simulink model "lab4_2"  (R2015a)
settings: Solver=ode5  StartTime=0.0  StopTime=inf  RelTol=1e-3
undefined symbols (not defined in the file or in its folder): National_Instruments, PCI
libraries: rtwinlib x2
settings Model: SimulationMode=external  ExtModeTrigDuration=10000  Creator=u_labelectro  LastModifiedBy=ARTURO
settings DebuggingCC: UnderspecifiedInitializationDetection=Classic  MergeDetectMultiDrivingBlocksExec=none  SolverPrmCheckMsg=warning  StateNameClashWarn=warning
settings HardwareCC: ProdBitPerLong=64  ProdBitPerPointer=64  ProdIntDivRoundTo=Zero  ProdEndianess=LittleEndian  ProdWordSize=64  ProdHWDeviceType=Intel->x86-64  TargetBitPerLong=64  TargetBitPerPointer=64  TargetIntDivRoundTo=Zero  TargetEndianess=LittleEndian  TargetWordSize=64  TargetHWDeviceType=Intel->x86-64
settings RTWCC: SystemTargetFile=rtwin.tlc  TemplateMakefile=rtwin.tmf  Description=Real-Time Windows Target  RTWCompilerOptimization=on
settings CodeAppCC: MaxIdLength=95
settings RTWinTargetCC: TargetPreCompLibLocation=C:\Program Files\MATLAB\MATLAB Production Server\R2015a\toolbox\sldrt\lib\win64

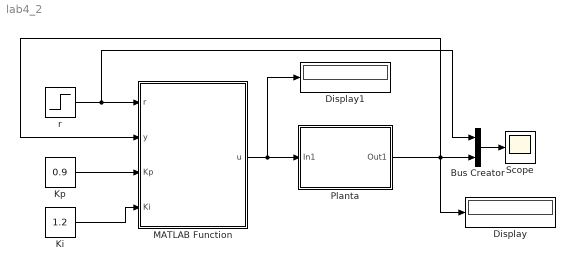
== system lab4_2 ==
  Bus Creator : BusCreator  Inputs=2
  Display : Display
  Display1 : Display
  Ki : Constant  Value=1.2
  Kp : Constant  Value=0.9
  MATLAB Function : MATLAB Function  TreatAsAtomicUnit=on
  Planta : Subsystem
  Scope : Scope
      settings: YMin=0  YMax=120  SaveName=signals
  r : Step  Time=0  After=60  SampleTime=0.01
  wires:
  Kp/1 -> MATLAB Function/3(Kp)
  Ki/1 -> MATLAB Function/4(Ki)
  r/1 -> Bus Creator/1, MATLAB Function/1(r)
  Planta/1(Out1) -> Bus Creator/2, Display/1, MATLAB Function/2(y)
  MATLAB Function/1(u) -> Display1/1, Planta/1(In1)
  Bus Creator/1 -> Scope/1

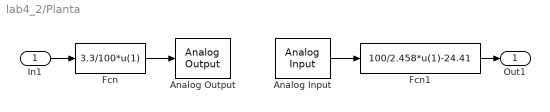
== system lab4_2/Planta ==
  In1 : Inport
  Analog Input : rtwinlib/Analog Input  SampleTime=0.01  MaxMissedTicks=10  ShowMissedTicks=off  YieldWhenWaiting=off  DrvName=National_Instruments/PCI-6229  DrvAddress=4294967295  DrvOptions=[0 0 0 0 0]  Channels=1  RangeMode=1  VoltRange=1  DataType=1
      settings: AttributesFormatString=National Instruments\nPCI-6229 [auto]
  Analog Output : rtwinlib/Analog Output  SampleTime=0.01  MaxMissedTicks=10  ShowMissedTicks=off  YieldWhenWaiting=off  DrvName=National_Instruments/PCI-6229  DrvAddress=4294967295  DrvOptions=[0 0 0 0 0]  Channels=1  RangeMode=1  VoltRange=1  InitialValue=[]  FinalValue=[]
      settings: AttributesFormatString=National Instruments\nPCI-6229 [auto]
  Fcn : Fcn  Expr=3.3/100*u(1)  SampleTime=0.01
  Fcn1 : Fcn  Expr=100/2.458*u(1)-24.41  SampleTime=0.01
  Out1 : Outport
  wires:
  Fcn/1 -> Analog Output/1
  In1/1 -> Fcn/1
  Fcn1/1 -> Out1/1
  Analog Input/1 -> Fcn1/1

== matlab function lab4_2/MATLAB Function ==
  data: r input; y input; Kp input; Ki input; u output
function u = controlador_PI(r,y,Kp,Ki)

T = 0.01;

persistent e_ant;
persistent u_ant;
persistent Int_ant;

if isempty(u_ant)
    u_ant = 0;
    e_ant = 0;
    Int_ant = 0;
end

e_act = r - y;

% Diferencias en retroceso
% Prop = (e_act - e_ant)*Kp;
% Int = e_act*Ki*T;
% u_act = u_ant + Prop + Int;
% Kp = 0.9, Ki = 1.2

% Aproximacion de Tustin
Prop = e_act*Kp;
%Der = Kd/T*(e_act - e_ant);
Int = e_act*T*Ki + Int_ant;
Int_ant = Int;
u_act = Prop + Int;
% Kp = 0.9, Ki = 1.2
% Kp = 0.5, Ki = 1


if (u_act<0)
    u_act = 0;
elseif (u_act>100)
    u_act = 100;
end

e_ant = e_act;
u_ant = u_act;
u = u_act;
end
